simulink model "pendulum_double_PID"  (R2024a)
settings: Solver=VariableStepAuto  StartTime=0.0  StopTime=500  RelTol=1e-3
values from neighbouring files (symbols this model uses):
  A0 = 0.032    [main.m]
  b1 = 0.3    [main.m]
  b2 = 0    [main.m]
  Cd = 1.2    [main.m]
  g = 9.8    [main.m]
  I = (m*l^2) / 3    (= 0.0416666666667)    [main.m]
  l = 0.5    [main.m]
  m = 0.5    [main.m]
  M = 1    [main.m]
  rho = 1.293    [main.m]
  theta0 = 30 * pi/180    (= 0.523598775598)    [main.m]
settings Model: Creator=yiming  LastModifiedBy=yiming

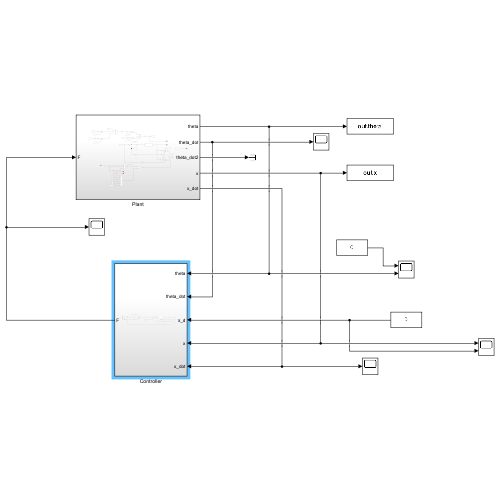
[thumbnail: Simulink's stored preview of the top-level diagram]
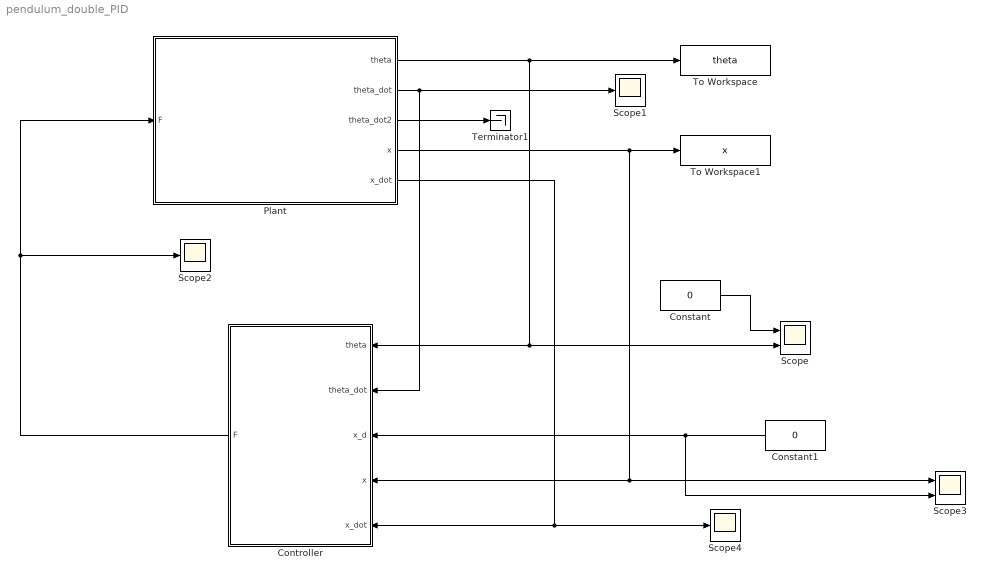
== system pendulum_double_PID ==
  Constant : Constant  Value=0
  Constant1 : Constant  Value=0
  Controller : Subsystem
  Plant : Subsystem
  Scope : Scope  NumInputPorts=2
  Scope1 : Scope
  Scope2 : Scope
  Scope3 : Scope  NumInputPorts=2
  Scope4 : Scope
  Terminator1 : Terminator
  To Workspace : ToWorkspace  VariableName=theta  SaveFormat=Timeseries  SampleTime=-1
  To Workspace1 : ToWorkspace  VariableName=x  SaveFormat=Timeseries  SampleTime=-1
  wires:
  Plant/1(theta) -> To Workspace/1, Scope/2, Controller/1(theta)
  Plant/3(theta_dot2) -> Terminator1/1
  Constant/1 -> Scope/1
  Controller/1(F) -> Scope2/1, Plant/1(F)
  Plant/2(theta_dot) -> Controller/2(theta_dot), Scope1/1
  Plant/4(x) -> Controller/4(x), Scope3/1, To Workspace1/1
  Plant/5(x_dot) -> Controller/5(x_dot), Scope4/1
  Constant1/1 -> Scope3/2, Controller/3(x_d)

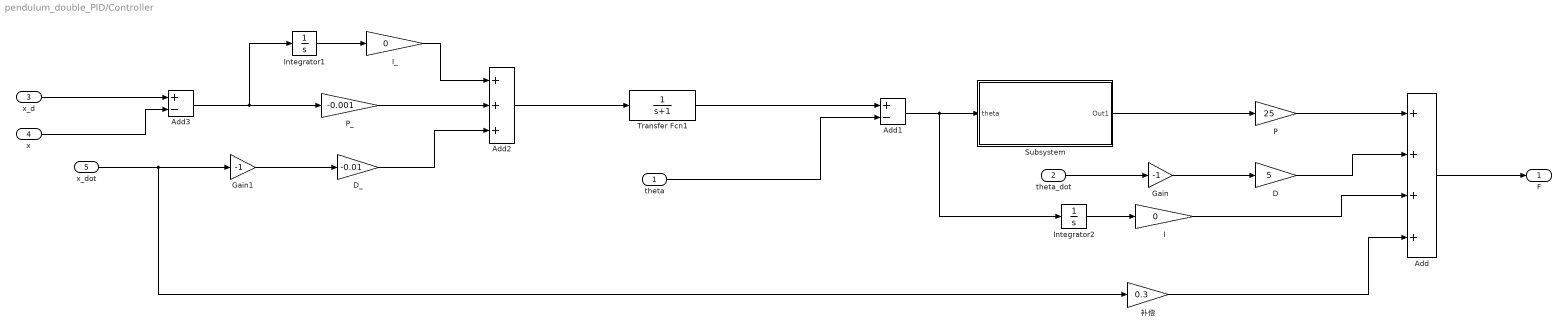
== system pendulum_double_PID/Controller ==
  theta : Inport
  theta_dot : Inport  Port=2
  x_d : Inport  Port=3
  x : Inport  Port=4
  x_dot : Inport  Port=5
  Add : Sum  Inputs=++++
  Add1 : Sum  Inputs=+-
  Add2 : Sum  Inputs=+++
  Add3 : Sum  Inputs=+-
  D : Gain  Gain=5
  D_ : Gain  Gain=-0.01
  Gain : Gain  Gain=-1
  Gain1 : Gain  Gain=-1
  I : Gain  Gain=0
  I_ : Gain  Gain=0
  Integrator1 : Integrator
  Integrator2 : Integrator
  P : Gain  Gain=25
  P_ : Gain  Gain=-0.001
  Subsystem : Subsystem
      settings: AttributesFormatString=保证角度值在正负180°之间
  Transfer Fcn1 : TransferFcn  Denominator=[1 1]
  补偿 : Gain  Gain=0.3
  F : Outport
  wires:
  P/1 -> Add/1
  Gain/1 -> D/1
  Add/1 -> F/1
  theta_dot/1 -> Gain/1
  theta/1 -> Add1/2
  Subsystem/1(Out1) -> P/1
  D/1 -> Add/2
  Gain1/1 -> D_/1
  Add3/1 -> Integrator1/1, P_/1
  x_dot/1 -> 补偿/1, Gain1/1
  Integrator1/1 -> I_/1
  I_/1 -> Add2/1
  P_/1 -> Add2/2
  D_/1 -> Add2/3
  x_d/1 -> Add3/1
  x/1 -> Add3/2
  补偿/1 -> Add/4
  Add1/1 -> Integrator2/1, Subsystem/1(theta)
  Integrator2/1 -> I/1
  I/1 -> Add/3
  Transfer Fcn1/1 -> Add1/1
  Add2/1 -> Transfer Fcn1/1

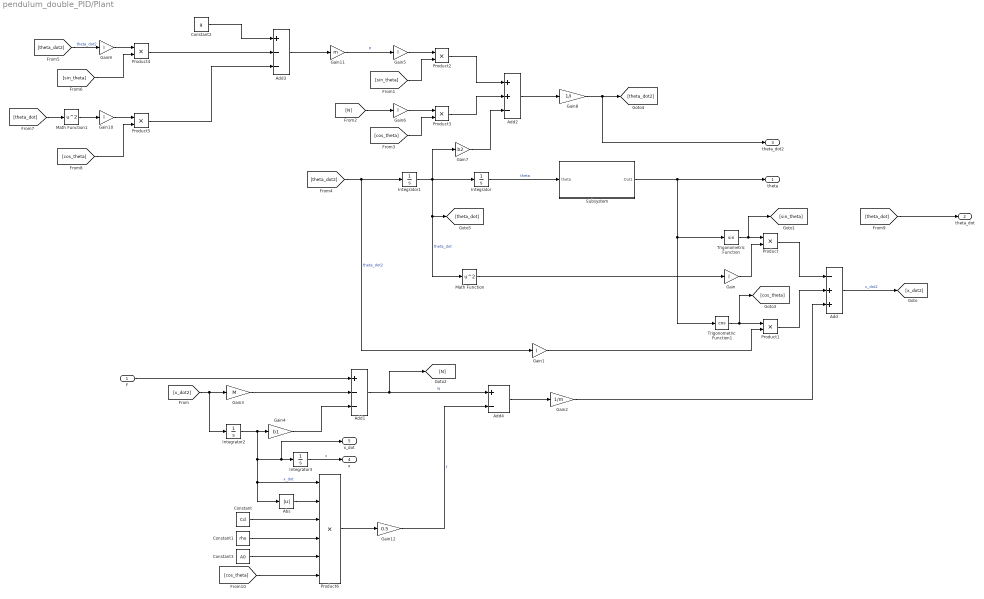
== system pendulum_double_PID/Plant ==
  F : Inport
  Abs : Abs  SaturateOnIntegerOverflow=off
  Add : Sum  Inputs=-++
  Add1 : Sum  Inputs=+--
  Add2 : Sum  Inputs=++-
  Add3 : Sum  Inputs=+--
  Add4 : Sum  Inputs=+-
  Constant : Constant  Value=Cd
  Constant1 : Constant  Value=rho
  Constant2 : Constant  Value=g
  Constant3 : Constant  Value=A0
  Gain{,1,5..6,9..10} (6 alike) : Gain  Gain=l
  Gain11 : Gain  Gain=m
  Gain12 : Gain  Gain=0.5
  Gain2 : Gain  Gain=1/m
  Gain3 : Gain  Gain=M
  Gain4 : Gain  Gain=b1
  Gain7 : Gain  Gain=b2
  Gain8 : Gain  Gain=1/I
  Integrator : Integrator  InitialCondition=theta0
  Integrator1 : Integrator
  Integrator2 : Integrator
  Integrator3 : Integrator
  Math Function : Math  Operator=square
  Math Function1 : Math  Operator=square
  Product{,1..5} (6 alike) : Product
  Product6 : Product  Inputs=6
  Subsystem : Subsystem
      settings: AttributesFormatString=保证角度值在正负180°之间
  Trigonometric Function : Trigonometry
  Trigonometric Function1 : Trigonometry  Operator=cos
  theta : Outport
  theta_dot : Outport  Port=2
  theta_dot2 : Outport  Port=3
  x : Outport  Port=4
  x_dot : Outport  Port=5
  wires:
  Integrator1/1 -> Gain7/1, Integrator/1, [theta_dot], Math Function/1  "theta_dot"
  Math Function/1 -> Gain/1
  Trigonometric Function/1 -> [sin_theta], Product/1
  Gain/1 -> Product/2
  [theta_dot2] -> Gain1/1, Integrator1/1  "theta_dot2"
  Trigonometric Function1/1 -> Product1/1, [cos_theta]
  Gain1/1 -> Product1/2
  Product1/1 -> Add/2
  Product/1 -> Add/1
  Add1/1 -> Add4/1, [N]  "N"
  Add/1 -> [x_dot2]  "x_dot2"
  Gain2/1 -> Add/3
  [x_dot2] -> Integrator2/1, Gain3/1
  Gain3/1 -> Add1/2
  Integrator2/1 -> Product6/1, Abs/1, x_dot/1, Integrator3/1, Gain4/1  "x_dot"
  Gain4/1 -> Add1/3
  Gain11/1 -> Gain5/1  "P"
  Gain5/1 -> Product2/1
  [sin_theta] -> Product2/2
  [N] -> Gain6/1
  Gain6/1 -> Product3/1
  [cos_theta] -> Product3/2
  Product2/1 -> Add2/1
  Product3/1 -> Add2/2
  Gain7/1 -> Add2/3
  Add2/1 -> Gain8/1
  Gain8/1 -> theta_dot2/1, [theta_dot2]
  [theta_dot2] -> Gain9/1  "theta_dot2"
  Gain9/1 -> Product4/1
  [sin_theta] -> Product4/2
  [theta_dot] -> Math Function1/1
  Math Function1/1 -> Gain10/1
  Gain10/1 -> Product5/1
  [cos_theta] -> Product5/2
  Product4/1 -> Add3/2
  Product5/1 -> Add3/3
  Constant2/1 -> Add3/1
  Add3/1 -> Gain11/1
  [theta_dot] -> theta_dot/1
  Integrator3/1 -> x/1  "x"
  Add4/1 -> Gain2/1
  Abs/1 -> Product6/2
  Constant/1 -> Product6/3
  Constant1/1 -> Product6/4
  [cos_theta] -> Product6/6
  Constant3/1 -> Product6/5
  Product6/1 -> Gain12/1
  Gain12/1 -> Add4/2  "f"
  F/1 -> Add1/1
  Integrator/1 -> Subsystem/1(theta)  "theta"
  Subsystem/1(Out1) -> Trigonometric Function1/1, Trigonometric Function/1, theta/1

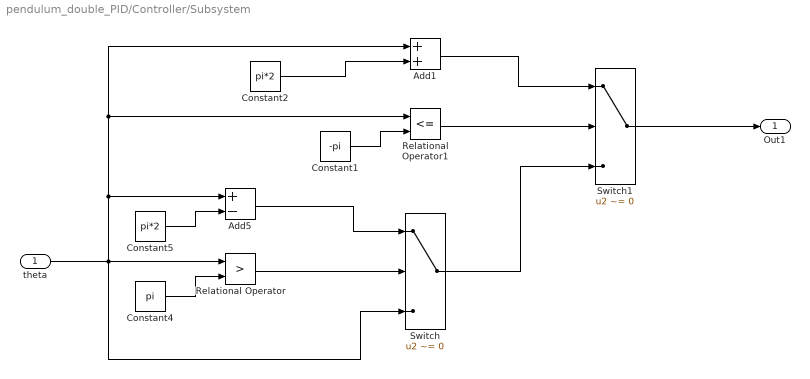
== system pendulum_double_PID/Controller/Subsystem ==
  theta : Inport
  Add1 : Sum
  Add5 : Sum  Inputs=+-
  Constant1 : Constant  Value=-pi
  Constant2 : Constant  Value=pi*2
  Constant4 : Constant  Value=pi
  Constant5 : Constant  Value=pi*2
  Relational Operator : RelationalOperator  Operator=>  OutDataTypeStr=boolean  RndMeth=Simplest  InputSameDT=off
  Relational Operator1 : RelationalOperator  Operator=<=  OutDataTypeStr=boolean  RndMeth=Simplest  InputSameDT=off
  Switch : Switch  Criteria=u2 ~= 0  SaturateOnIntegerOverflow=off  InputSameDT=off
      settings: AttributesFormatString=保证角度值不越过+180°
  Switch1 : Switch  Criteria=u2 ~= 0  SaturateOnIntegerOverflow=off  InputSameDT=off
      settings: AttributesFormatString=保证角度值不越过-180°
  Out1 : Outport
  wires:
  Constant5/1 -> Add5/2
  Constant4/1 -> Relational Operator/2
  Relational Operator/1 -> Switch/2
  theta/1 -> Relational Operator/1, Switch/3, Add1/1, Relational Operator1/1, Add5/1
  Add5/1 -> Switch/1
  Constant1/1 -> Relational Operator1/2
  Relational Operator1/1 -> Switch1/2
  Constant2/1 -> Add1/2
  Add1/1 -> Switch1/1
  Switch/1 -> Switch1/3
  Switch1/1 -> Out1/1

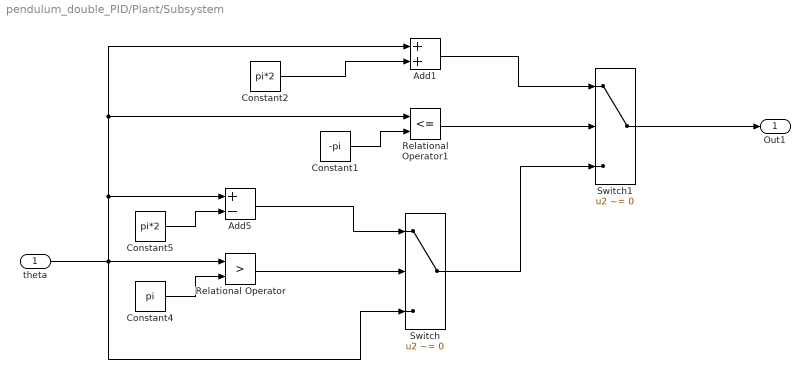
== system pendulum_double_PID/Plant/Subsystem ==
  theta : Inport
  Add1 : Sum
  Add5 : Sum  Inputs=+-
  Constant1 : Constant  Value=-pi
  Constant2 : Constant  Value=pi*2
  Constant4 : Constant  Value=pi
  Constant5 : Constant  Value=pi*2
  Relational Operator : RelationalOperator  Operator=>  OutDataTypeStr=boolean  RndMeth=Simplest  InputSameDT=off
  Relational Operator1 : RelationalOperator  Operator=<=  OutDataTypeStr=boolean  RndMeth=Simplest  InputSameDT=off
  Switch : Switch  Criteria=u2 ~= 0  SaturateOnIntegerOverflow=off  InputSameDT=off
      settings: AttributesFormatString=保证角度值不越过+180°
  Switch1 : Switch  Criteria=u2 ~= 0  SaturateOnIntegerOverflow=off  InputSameDT=off
      settings: AttributesFormatString=保证角度值不越过-180°
  Out1 : Outport
  wires:
  Constant5/1 -> Add5/2
  Constant4/1 -> Relational Operator/2
  Relational Operator/1 -> Switch/2
  theta/1 -> Relational Operator/1, Switch/3, Add1/1, Relational Operator1/1, Add5/1
  Add5/1 -> Switch/1
  Constant1/1 -> Relational Operator1/2
  Relational Operator1/1 -> Switch1/2
  Constant2/1 -> Add1/2
  Add1/1 -> Switch1/1
  Switch/1 -> Switch1/3
  Switch1/1 -> Out1/1
